simulink model "SingleBuckLQILoadChange"  (R2018b)
settings: Solver=ode23tb  StartTime=0.0  StopTime=1  RelTol=1e-3
undefined symbols (not defined in the file): C, K, Ki, L, R, rL
libraries: powerlib x12, powerlib_meascontrol x1
settings Model: Creator=Charles-Spencer  LastModifiedBy=Charles-Spencer

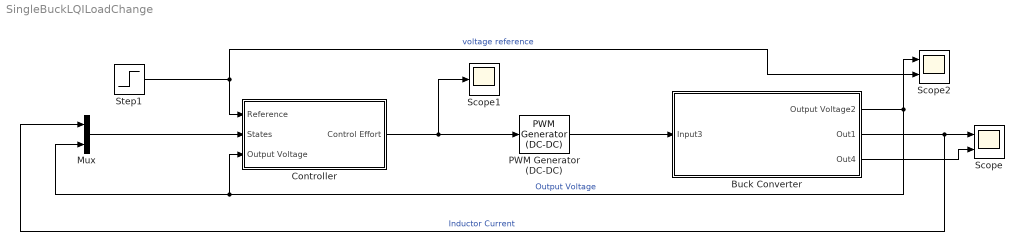
== system SingleBuckLQILoadChange ==
  Buck Converter : Subsystem
  Controller : Subsystem
  Mux : Mux  Inputs=2
  PWM Generator (DC-DC) : powerlib_meascontrol/Pulse & Signal Generators/PWM Generator (DC-DC)  Fsw=fsw  Ts=0
      settings: SourceProductName=Simscape Electrical
  Scope : Scope  NumInputPorts=2
  Scope1 : Scope
  Scope2 : Scope  NumInputPorts=2
  Step1 : Step  Before=48  After=48  SampleTime=0
  wires:
  PWM Generator (DC-DC)/1 -> Buck Converter/1(Input3)
  Buck Converter/1(Output Voltage2) -> Scope2/1, Controller/3(Output Voltage), Mux/2  "Output Voltage"
  Controller/1(Control Effort) -> Scope1/1, PWM Generator (DC-DC)/1
  Mux/1 -> Controller/2(States)
  Step1/1 -> Controller/1(Reference), Scope2/2  "voltage reference"
  Buck Converter/2(Out1) -> Mux/1, Scope/1  "Inductor Current"
  Buck Converter/3(Out4) -> Scope/2

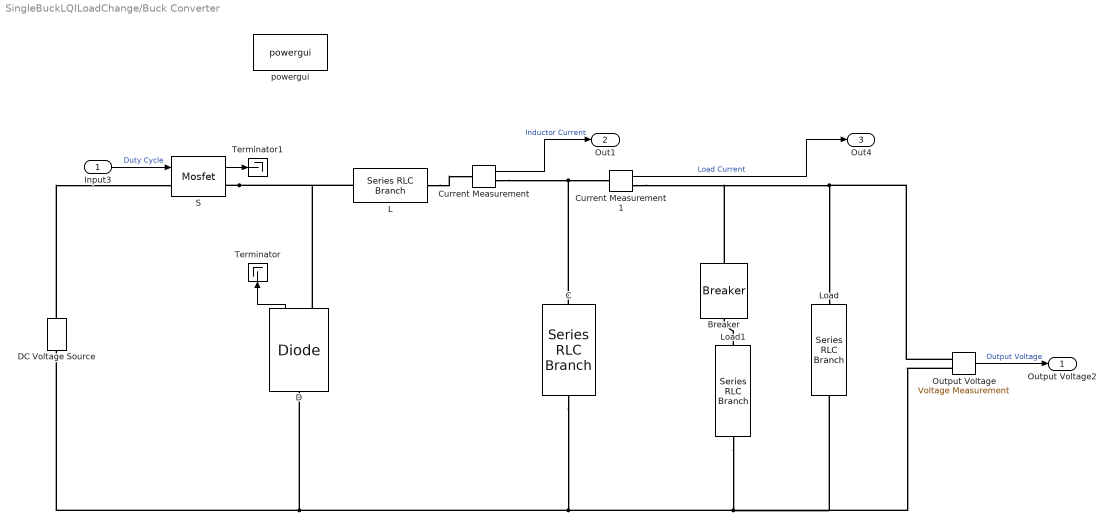
== system SingleBuckLQILoadChange/Buck Converter ==
  Input3 : Inport
  Breaker : powerlib/Elements/Breaker  InitialState=0  SwitchingTimes=0.5  External=off  BreakerResistance=0.01  SnubberResistance=1e6  SnubberCapacitance=inf  Measurements=None  MoreParameters=on  NoBreakLoop=off
      settings: SourceProductName=Simscape Power Systems
  C : powerlib/Elements/Series RLC Branch  LConnTagsString=__new0  RConnTagsString=__new0  BranchType=C  Resistance=1  Inductance=1e-3  SetiL0=off  InitialCurrent=0  Capacitance=C  Setx0=off  InitialVoltage=0  Measurements=None
      settings: SourceProductName=Simscape Electrical
  Current Measurement : powerlib/Measurements/Current Measurement  PhasorSimulation=off  OutputType=Complex  PSBequivalent=0
      settings: SourceProductName=Simscape Electrical
  Current Measurement1 : powerlib/Measurements/Current Measurement  PhasorSimulation=off  OutputType=Complex  PSBequivalent=0
      settings: SourceProductName=Simscape Electrical
  D : powerlib/Power Electronics/Diode  Ron=0.0001  Lon=0  Vf=0  IC=0  UseSnubber=off  Rs=5000  Cs=250e-9  Measurements=on
      settings: SourceProductName=Simscape Electrical
  DC Voltage Source : powerlib/Electrical Sources/DC Voltage Source  Amplitude=100  Measurements=None
  L : powerlib/Elements/Series RLC Branch  LConnTagsString=__new0  RConnTagsString=__new0  BranchType=RL  Resistance=rL  Inductance=L  SetiL0=off  InitialCurrent=0  Capacitance=1e-6  Setx0=off  InitialVoltage=0  Measurements=None
      settings: SourceProductName=Simscape Electrical
  Load : powerlib/Elements/Series RLC Branch  LConnTagsString=__new0  RConnTagsString=__new0  BranchType=R  Resistance=R  Inductance=1e-3  SetiL0=off  InitialCurrent=0  Capacitance=1e-6  Setx0=off  InitialVoltage=0  Measurements=None
      settings: SourceProductName=Simscape Electrical
  Load1 : powerlib/Elements/Series RLC Branch  LConnTagsString=__new0  RConnTagsString=__new0  BranchType=R  Resistance=2*R  Inductance=1e-3  SetiL0=off  InitialCurrent=0  Capacitance=1e-6  Setx0=off  InitialVoltage=0  Measurements=None
      settings: SourceProductName=Simscape Electrical
  Output Voltage : powerlib/Measurements/Voltage Measurement  PhasorSimulation=off  OutputType=Complex  PSBequivalent=0
      settings: SourceProductName=Simscape Electrical
  S : powerlib/Power Electronics/Mosfet  Ron=0.001  Lon=0  Rd=0.0001  Vfd=0  IC=0  Rs=1e5  Cs=inf  Measurements=on
      settings: SourceProductName=Simscape Electrical
  Terminator : Terminator
  Terminator1 : Terminator
  powergui : powerlib/powergui  Priority=1  SimulationMode=Continuous  SampleTime=50e-8  frequency=60  Iterations=50  frequencyindice=0  Pbase=100e6  ErrMax=1e-4  UnitsV=kV  UnitsW=MW  buscounter=0  FunctionMessages=off  echomessages=off  EnableUseOfTLC=off  CurrentSourceSwitches=off  DisableSnubberDevices=off  DisableRonSwitches=off  DisableVfSwitches=off  DisplayEquations=off  SolverType=Tustin/Backward Euler (TBE)  Interpol=off  ExternalGateDelay=off  methode=off  Ts=100  x0status=blocks  SPID=on  SwTol=0  HookPort=off  RestoreLinks=warning  ResistiveCurrentMeasurement=off  Frange=[0:2:500]  Ylog=off  Xlog=on  ShowGrid=off  save=off  variable=ZData  structure=0  ZoomFFT=off  StartTime=0.0  cycles=1  DisplayStyle=1  fundamental=60  FreqAxis=off  MaxFrequency=1000  frequencyindicesteady=1  RmsSteady=1  display=off
  Output Voltage2 : Outport
  Out1 : Outport  Port=2
  Out4 : Outport  Port=3
  wires:
  Current Measurement1/1 -> Out4/1  "Load Current"
  Output Voltage/1 -> Output Voltage2/1  "Output Voltage"
  Current Measurement/1 -> Out1/1  "Inductor Current"
  Input3/1 -> S/1  "Duty Cycle"
  D/1 -> Terminator/1
  S/1 -> Terminator1/1
  connections:
  Current Measurement/RConn1 -- C/LConn1 -- Current Measurement1/LConn1
  C/RConn1 -- Load1/RConn1 -- Output Voltage/LConn2 -- Load/RConn1 -- DC Voltage Source/LConn1 -- D/LConn1
  S/RConn1 -- L/LConn1 -- D/RConn1
  L/RConn1 -- Current Measurement/LConn1
  DC Voltage Source/RConn1 -- S/LConn1
  Output Voltage/LConn1 -- Current Measurement1/RConn1 -- Breaker/RConn1 -- Load/LConn1
  Load1/LConn1 -- Breaker/LConn1

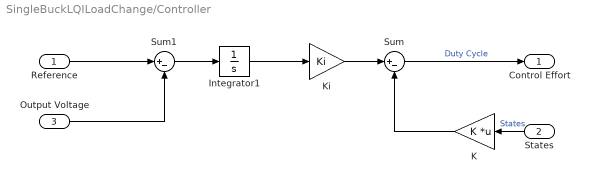
== system SingleBuckLQILoadChange/Controller ==
  Reference : Inport
  States : Inport  Port=2
  Output Voltage : Inport  Port=3
  Integrator1 : Integrator
  K : Gain  Gain=K  Multiplication=Matrix(K*u)
  Ki : Gain  Gain=Ki
  Sum : Sum  Inputs=|+-
  Sum1 : Sum  Inputs=|+-
  Control Effort : Outport
  wires:
  Integrator1/1 -> Ki/1
  Reference/1 -> Sum1/1
  Sum/1 -> Control Effort/1  "Duty Cycle"
  States/1 -> K/1  "States"
  Sum1/1 -> Integrator1/1
  Output Voltage/1 -> Sum1/2
  Ki/1 -> Sum/1
  K/1 -> Sum/2
